simulink model "evaporator"  (R2019a)
settings: Solver=VariableStepAuto  StartTime=0.0  StopTime=10.0  RelTol=1e-3
settings Model: Creator=amah2  LastModifiedBy=amah2

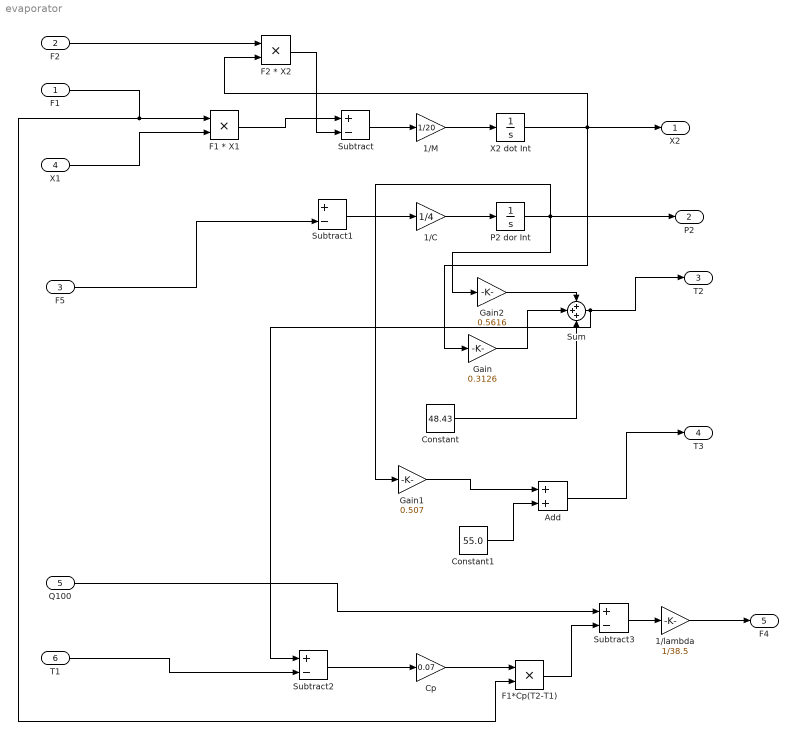
== system evaporator ==
  F1 : Inport
  F2 : Inport  Port=2
  F5 : Inport  Port=3
  X1 : Inport  Port=4
  Q100 : Inport  Port=5
  T1 : Inport  Port=6
  1/C : Gain  Gain=1/4
  1/M : Gain  Gain=1/20
  1/lambda : Gain  Gain=1/38.5
  Add : Sum
  Constant : Constant  Value=48.43
  Constant1 : Constant  Value=55.0
  Cp : Gain  Gain=0.07
  F1 * X1 : Product
  F1*Cp(T2-T1) : Product
  F2 * X2 : Product
  Gain : Gain  Gain=0.3126
  Gain1 : Gain  Gain=0.507
  Gain2 : Gain  Gain=0.5616
  P2 dor Int : Integrator
  Subtract{,1..3} (4 alike) : Sum  Inputs=+-
  Sum : Sum  Inputs=+++
  X2 dot Int : Integrator
  X2 : Outport
  "P2 " : Outport  Port=2
  "T2 " : Outport  Port=3
  "T3 " : Outport  Port=4
  "F4 " : Outport  Port=5
  wires:
  X2 dot Int/1 -> Gain/1, X2/1, F2 * X2/2
  1/M/1 -> X2 dot Int/1
  F1/1 -> F1 * X1/1, F1*Cp(T2-T1)/2
  X1/1 -> F1 * X1/2
  Subtract/1 -> 1/M/1
  F1 * X1/1 -> Subtract/1
  F2/1 -> F2 * X2/1
  F2 * X2/1 -> Subtract/2
  1/C/1 -> P2 dor Int/1
  Subtract1/1 -> 1/C/1
  F5/1 -> Subtract1/2
  P2 dor Int/1 -> Gain2/1, Gain1/1, "P2 "/1
  Sum/1 -> Subtract2/1, "T2 "/1
  Gain2/1 -> Sum/1
  Gain/1 -> Sum/2
  Constant/1 -> Sum/3
  Constant1/1 -> Add/2
  Gain1/1 -> Add/1
  Add/1 -> "T3 "/1
  Subtract3/1 -> 1/lambda/1
  1/lambda/1 -> "F4 "/1
  Q100/1 -> Subtract3/1
  F1*Cp(T2-T1)/1 -> Subtract3/2
  Cp/1 -> F1*Cp(T2-T1)/1
  Subtract2/1 -> Cp/1
  T1/1 -> Subtract2/2
